simulink library "N7_6lib"  (R2016a)
settings: Solver=ode45  StartTime=0.0  StopTime=10.0  RelTol=1e-3
settings Model: Creator=Kayab  LastModifiedBy=Kayab
settings DataIOCC: LimitDataPoints=on
settings DebuggingCC: AllowSymbolicDim=off

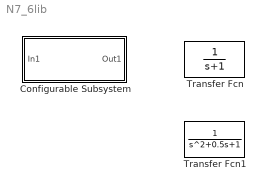
== system N7_6lib ==
  Configurable Subsystem : Subsystem  BlockChoice=Transfer Fcn
      settings: TemplateBlock=self  MemberBlocks=Transfer Fcn,Transfer Fcn1
  Transfer Fcn : TransferFcn  Denominator=[1 1]
  Transfer Fcn1 : TransferFcn  Denominator=[1 0.5 1]

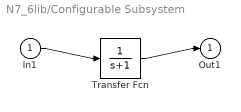
== system N7_6lib/Configurable Subsystem ==
  In1 : Inport
  Transfer Fcn : TransferFcn  Denominator=[1 1]
  Out1 : Outport
  wires:
  In1/1 -> Transfer Fcn/1
  Transfer Fcn/1 -> Out1/1
